simulink model "problem2"  (R2024b)
settings: Solver=VariableStepAuto  StartTime=0.0  StopTime=1000.0  RelTol=1e-3
settings Model: Creator=djd14  LastModifiedBy=djd14

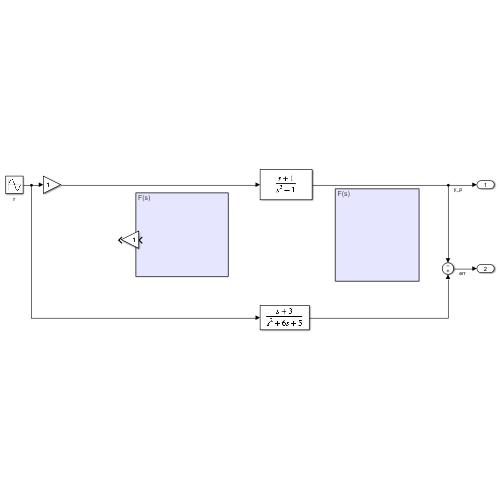
[thumbnail: Simulink's stored preview of the top-level diagram]
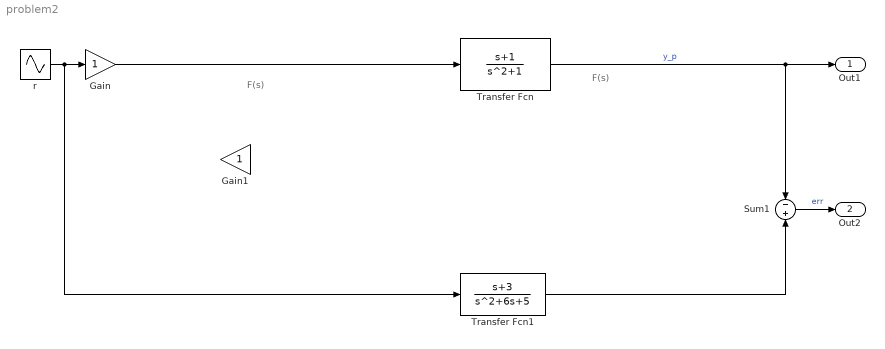
== system problem2 ==
  note: F(s)
  note: F(s)
  Gain : Gain
  Gain1 : Gain
  Sum1 : Sum  Inputs=-|+
  Transfer Fcn : TransferFcn  Numerator=[1 1]  Denominator=[1 0 1]
  Transfer Fcn1 : TransferFcn  Numerator=[1 3]  Denominator=[1 6 5]
  r : Sin  Amplitude=2  SampleTime=0
  Out1 : Outport
  Out2 : Outport  Port=2
  wires:
  r/1 -> Transfer Fcn1/1, Gain/1
  Gain/1 -> Transfer Fcn/1
  Transfer Fcn/1 -> Sum1/1, Out1/1  "y_p"
  Transfer Fcn1/1 -> Sum1/2
  Sum1/1 -> Out2/1  "err"
